simulink model "InjCtl_qCo"  (R2018a)
settings: configuration reference "cs_ert" (kept outside this file)
settings Model: DataDictionary=InjCtl_qCo.sldd  Creator=zhoutinglin  LastModifiedBy=zhoutinglin

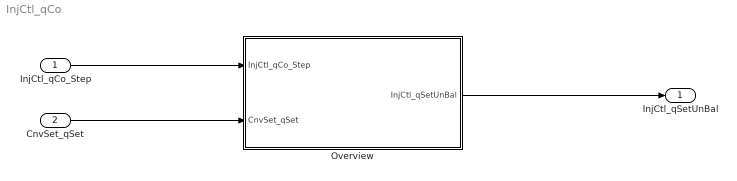
== system InjCtl_qCo ==
  InjCtl_qCo_Step : Inport  OutputFunctionCall=on
  CnvSet_qSet : Inport  Description=Injection quantity current path  Port=2  OutMin=-319  OutMax=319  OutDataTypeStr=InjMass  Unit=mg/hub  PortDimensions=[1 1]
  Overview : Subsystem
  InjCtl_qSetUnBal : Outport  Description=Torque generating engine fuel injection quantity  OutMin=-319  OutMax=319  OutDataTypeStr=InjMass  Unit=mg/hub  PortDimensions=[1 1]
  wires:
  InjCtl_qCo_Step/1 -> Overview/1(InjCtl_qCo_Step)
  CnvSet_qSet/1 -> Overview/2(CnvSet_qSet)
  Overview/1(InjCtl_qSetUnBal) -> InjCtl_qSetUnBal/1

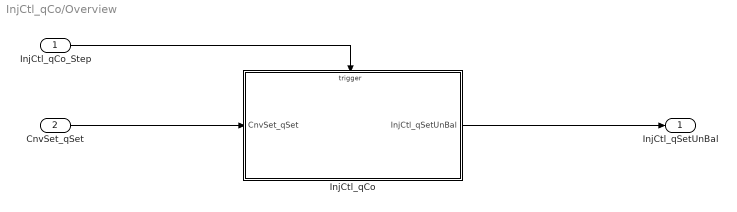
== system InjCtl_qCo/Overview ==
  InjCtl_qCo_Step : Inport
  CnvSet_qSet : Inport  Port=2
  InjCtl_qCo : Subsystem
  InjCtl_qSetUnBal : Outport
  wires:
  CnvSet_qSet/1 -> InjCtl_qCo/1(CnvSet_qSet)
  InjCtl_qCo/1(InjCtl_qSetUnBal) -> InjCtl_qSetUnBal/1
  InjCtl_qCo_Step/1 -> InjCtl_qCo/Trigger

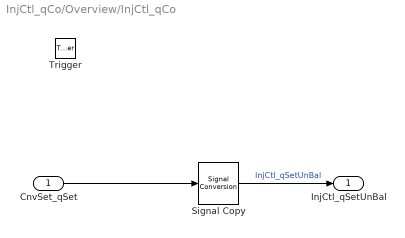
== system InjCtl_qCo/Overview/InjCtl_qCo ==
  CnvSet_qSet : Inport
  Trigger : TriggerPort  TriggerType=function-call  VariantControl=Variant  PortDimensions=1
  Signal Copy : SignalConversion  OverrideOpt=off
  InjCtl_qSetUnBal : Outport
  wires:
  Signal Copy/1 -> InjCtl_qSetUnBal/1  "InjCtl_qSetUnBal"
  CnvSet_qSet/1 -> Signal Copy/1
